simulink model "week1_6"  (R2020b)
settings: Solver=VariableStepAuto  StartTime=0.0  StopTime=10.0  RelTol=1e-3
settings Model: Creator=Lenovo  LastModifiedBy=Lenovo

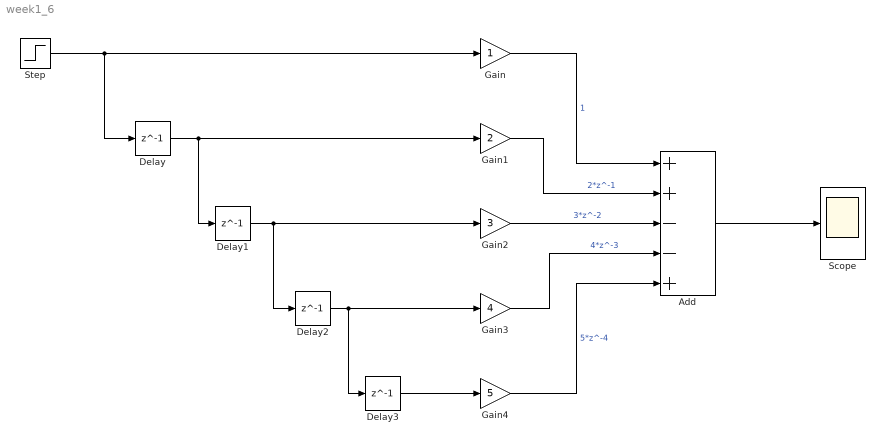
== system week1_6 ==
  Add : Sum  Inputs=++--+
  Delay{,1..3} (4 alike) : Delay  DelayLength=1  InitialCondition=0
  Gain : Gain
  Gain1 : Gain  Gain=2
  Gain2 : Gain  Gain=3
  Gain3 : Gain  Gain=4
  Gain4 : Gain  Gain=5
  Scope : Scope
  Step : Step  SampleTime=0
  wires:
  Step/1 -> Delay/1, Gain/1
  Gain/1 -> Add/1  "1"
  Add/1 -> Scope/1
  Delay/1 -> Delay1/1, Gain1/1
  Gain1/1 -> Add/2  "2*z^-1"
  Delay1/1 -> Delay2/1, Gain2/1
  Gain2/1 -> Add/3  "3*z^-2"
  Delay2/1 -> Delay3/1, Gain3/1
  Gain3/1 -> Add/4  "4*z^-3"
  Delay3/1 -> Gain4/1
  Gain4/1 -> Add/5  "5*z^-4"
